simulink model "Propellers"  (R2018b)
settings: Solver=VariableStepAuto  StartTime=0.0  StopTime=10.0  RelTol=1e-3
settings Model: Creator=karlemstrand  LastModifiedBy=karlemstrand

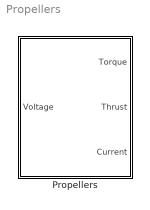
== system Propellers ==
  Propellers : MATLAB Function  TreatAsAtomicUnit=on

== matlab function Propellers/Propellers ==
  data: Voltage input; Torque output; Thrust output; Current output
function [Torque, Thrust, Current] = fcn(Voltage)
RPM = [0 0 0 0];
Torque = [0 0 0 0];
Thrust = [0 0 0 0];
Current = [0 0 0 0];

for i = 1 : 4
    RPM(i) = -2.6931 * Voltage(i)^3 + 1400 * Voltage(i);
    % From propeller lec
    CoefOfThrust = 2*10^-15 * RPM(i)^3 - 4*10^-11 * RPM(i)^2 + 3*10^-7 * RPM(i) + 0.1013;
    Thrust(i) = CoefOfThrust * 1.225 * (RPM(i) / 60)^2 * 0.2^4;
    Torque(i) = 4*10^-14 * RPM(i)^3 + 8*10^-12 * RPM(i)^2 + 3*10^-6 * RPM(i);
    Current(i) = 1400 * Torque(i);
end
